simulink model "fmcw_range_model"  (R2024b)
settings: Solver=FixedStepDiscrete  StartTime=0.0  StopTime=10e-6  FixedStep=5e-9  RelTol=1e-3
undefined symbols (not defined in the file): physconst
libraries: phasedenvlib x2, phaseddetectlib x1, phasedwavlib x1
settings Model: Creator=lloyd  LastModifiedBy=lloyd

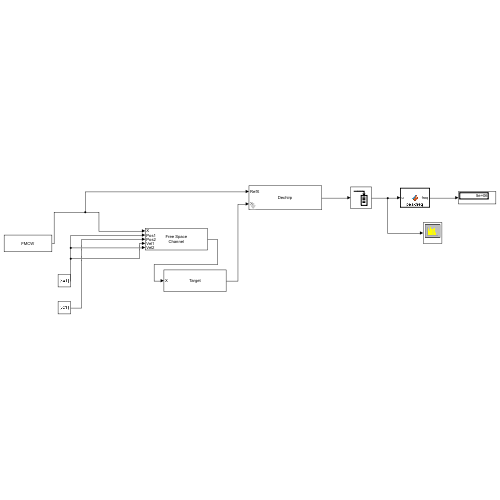
[thumbnail: Simulink's stored preview of the top-level diagram]
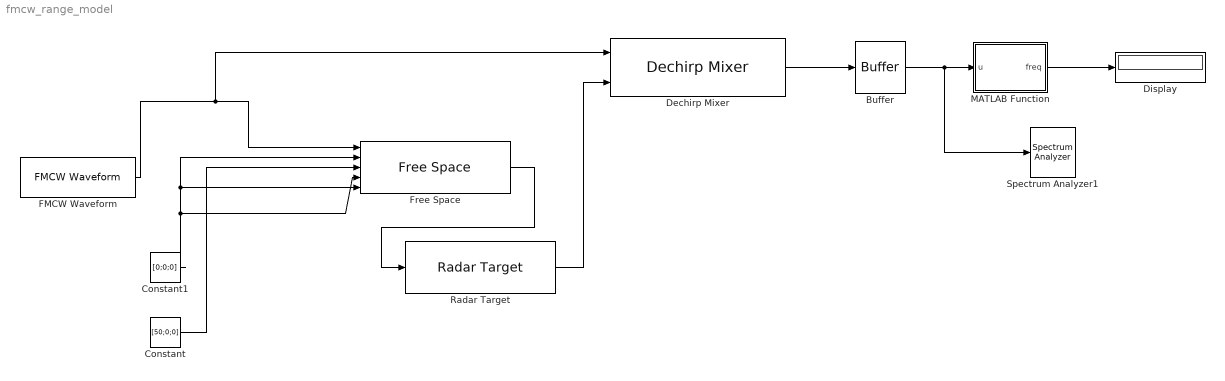
== system fmcw_range_model ==
  Buffer : Buffer  N=2000  OutputFrames=off
  Constant : Constant  Value=[50;0;0]
  Constant1 : Constant  Value=[0;0;0]
  Dechirp Mixer : phaseddetectlib/Dechirp Mixer
  Display : Display
  FMCW Waveform : phasedwavlib/FMCW Waveform  SampleRate=200e6  SweepTime=10e-6  SweepBandwidth=150e6  SweepDirection=Up  SweepInterval=Positive  OutputFormat=Samples  NumSamples=100  NumSweeps=1  SimulateUsing=Interpreted execution
  Free Space : phasedenvlib/Free Space  PropagationSpeed=3e8  OperatingFrequency=77e9  TwoWayPropagation=on  SampleRateFromInputCheckbox=on  SampleRate=1e6  MaximumDistanceSource=Property  MaximumDistance=500  MaximumNumInputSamplesSource=Auto  MaximumNumInputSamples=1000  SimulateUsing=Interpreted execution
  MATLAB Function : MATLAB Function  TreatAsAtomicUnit=on
  Radar Target : phasedenvlib/Radar Target  EnablePolarization=off  Mode=Monostatic  MeanRCSSource=Property  ScatteringMatrixSource=Property  MeanRCS=10  ScatteringMatrix=eye( 2 )  Model=Nonfluctuating  PropagationSpeed=physconst( 'LightSpeed' )  OperatingFrequency=77e9  SeedSource=Auto  Seed=0  SimulateUsing=Interpreted execution
  Spectrum Analyzer1 : SpectrumAnalyzer  WindowPosition=[368.000000,182.000000,800.000000,500.000000,]  Visible=on  ScopeFrameLocation=window  WindowInvariantSamplesPerUpdate=on  Span=200000000.00000003  StartFrequency=-100000000.00000001  StopFrequency=100000000.00000001  YLimits=[-221.75411698,-105.57771302]
  wires:
  FMCW Waveform/1 -> Dechirp Mixer/1, Free Space/1
  Constant1/1 -> Free Space/2, Free Space/5, Free Space/4
  Constant/1 -> Free Space/3
  Radar Target/1 -> Dechirp Mixer/2
  Free Space/1 -> Radar Target/1
  Dechirp Mixer/1 -> Buffer/1
  Buffer/1 -> Spectrum Analyzer1/1, MATLAB Function/1(u)
  MATLAB Function/1(freq) -> Display/1

== matlab function fmcw_range_model/MATLAB Function ==
  data: u input; freq output
function freq = peakfreq(u)
    Fs = 200e6;
    N = length(u);
    X = abs(fft(u));
    [~, idx] = max(X(1:floor(N/2)));
    freq = (idx-1) * (Fs/N);
end
